simulink model "SimulinkModel"  (R2025b)
settings: Solver=VariableStepAuto  StartTime=0.0  StopTime=90  FixedStep=0.10  MaxStep=0.1  MinStep=0.01  RelTol=0.5e-5  AbsTol=1e-5
values from neighbouring files (symbols this model uses):
  clock_drift_rate = 0.5    [run_simulink_batch.m]
  initial_q_IB = mission.Satellite.q0    [run_simulink_batch.m]
  nav_mekf_initial_P = [1e-2; 1e-2; 1e-2]    [run_simulink_batch.m]
  pod_kf_initial_P = [1e2; 1e2; 1e2; 1e2; 1e2; 1e2]    [run_simulink_batch.m]
  R_mag = diag([1; 2; 3])    [run_simulink_batch.m]
  R_sun = diag([1; 2; 3])    [run_simulink_batch.m]
  s = struct()    [applySensorNoise.m]
  w_earth = [0; 0; 7.2921159 * 10^(-5)]    [run_simulink_batch.m]
undefined symbols (not defined in the file or in its folder): accelCorrectionInterval, baroCorrectionInterval, deg, gpsCorrectionInterval, IAU, IMUPropInterval, magCorrectionInterval, R_vec, rad, WMM2025
libraries: aerolibtransform2 x11, matrix_library x6, vrlib x3, aerolibgravity2 x3, aerolibconvert2 x2, aerolibsatdyn x1, aerolibutil x1, aerolibnav x1
(part 2 of 2)

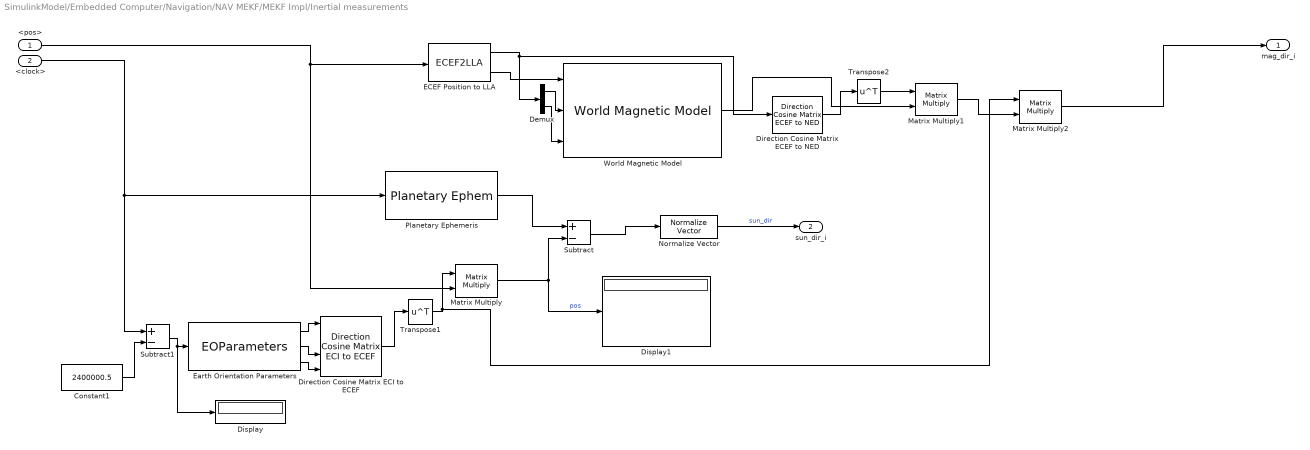
== system SimulinkModel/Embedded Computer/Navigation/NAV MEKF/MEKF Impl/Inertial measurements ==
  <pos> : Inport
  <clock> : Inport  Port=2
  Constant1 : Constant  Value=2400000.5
  Demux : Demux  Outputs=2
  Direction Cosine Matrix ECEF to NED : aerolibtransform2/Direction Cosine Matrix ECEF to NED
  Direction Cosine Matrix ECI to ECEF : aerolibtransform2/Direction Cosine Matrix ECI to ECEF  red=IAU-2000/2006  year=mission.StartDate.Year  month=January  day=1  hour=12  min=0  sec=0  deltaT=None  errorflag=Error  extraparamflag=on
      settings: AttributesFormatString=%<red>
  Display : Display
  Display1 : Display
  ECEF Position to LLA : ECEF2LLA
  Earth Orientation Parameters : EOParameters
  Matrix Multiply : Product  Multiplication=Matrix(*)
  Matrix Multiply1 : Product  Multiplication=Matrix(*)
  Matrix Multiply2 : Product  Multiplication=Matrix(*)
  Normalize Vector : vrlib/Utilities/Normalize Vector  maxzero=0
  Planetary Ephemeris : PlanetaryEphem  units=m,m/s  target=Sun  outputVelocity=off
  Subtract : Sum  Inputs=+-
  Subtract1 : Sum  Inputs=+-
  Transpose1 : Math  Operator=transpose
  Transpose2 : Math  Operator=transpose
  World Magnetic Model : aerolibgravity2/World Magnetic Model  model=WMM2025 (2025-2030)  customFile='WMM2025.COF'  units=Metric (MKS)  time_in=off  month=January  day=1  year=2025  action=Error  h_out=off  dec_out=off  inc_out=off  ti_out=off
  mag_dir_i : Outport
  sun_dir_i : Outport  Port=2
  wires:
  World Magnetic Model/1 -> Matrix Multiply1/2
  <pos>/1 -> Matrix Multiply/2, ECEF Position to LLA/1
  Direction Cosine Matrix ECI to ECEF/1 -> Transpose1/1
  Earth Orientation Parameters/3 -> Direction Cosine Matrix ECI to ECEF/4
  Subtract1/1 -> Display/1, Earth Orientation Parameters/1
  ECEF Position to LLA/1 -> Direction Cosine Matrix ECEF to NED/1, Demux/1
  <clock>/1 -> Planetary Ephemeris/1, Subtract1/1
  Demux/2 -> World Magnetic Model/3
  ECEF Position to LLA/2 -> World Magnetic Model/1
  Earth Orientation Parameters/2 -> Direction Cosine Matrix ECI to ECEF/3
  Earth Orientation Parameters/1 -> Direction Cosine Matrix ECI to ECEF/1
  Transpose1/1 -> Matrix Multiply2/1, Matrix Multiply/1
  Direction Cosine Matrix ECEF to NED/1 -> Transpose2/1
  Transpose2/1 -> Matrix Multiply1/1
  Subtract/1 -> Normalize Vector/1
  Constant1/1 -> Subtract1/2
  Matrix Multiply/1 -> Subtract/2, Display1/1  "pos"
  Demux/1 -> World Magnetic Model/2
  Planetary Ephemeris/1 -> Subtract/1
  Matrix Multiply2/1 -> mag_dir_i/1
  Matrix Multiply1/1 -> Matrix Multiply2/2
  Normalize Vector/1 -> sun_dir_i/1  "sun_dir"

== system SimulinkModel/Embedded Computer/Navigation/NAV MEKF/MEKF Impl/Mag Update ==
  oldState : Inport
  oldP : Inport  Port=2
  <mag> : Inport  Port=3
  mag_i : Inport  Port=4
  Constant : Constant  Value=R_mag
  MATLAB Function : MATLAB Function  TreatAsAtomicUnit=on
  state : Outport
  P : Outport  Port=2
  wires:
  oldState/1 -> MATLAB Function/1(oldState)
  MATLAB Function/1(state) -> state/1
  MATLAB Function/2(P) -> P/1
  oldP/1 -> MATLAB Function/2(oldP)
  <mag>/1 -> MATLAB Function/3(sens)
  Constant/1 -> MATLAB Function/5(R)
  mag_i/1 -> MATLAB Function/4(mag_i)

== system SimulinkModel/Embedded Computer/Navigation/NAV MEKF/MEKF Impl/Sun Update ==
  oldState : Inport
  oldP : Inport  Port=2
  <sun> : Inport  Port=3
  sun_i : Inport  Port=4
  Constant : Constant  Value=R_sun
  MATLAB Function : MATLAB Function  TreatAsAtomicUnit=on
  state : Outport
  P : Outport  Port=2
  wires:
  oldState/1 -> MATLAB Function/1(oldState)
  MATLAB Function/1(state) -> state/1
  MATLAB Function/2(P) -> P/1
  oldP/1 -> MATLAB Function/2(oldP)
  <sun>/1 -> MATLAB Function/3(sens)
  Constant/1 -> MATLAB Function/5(R)
  sun_i/1 -> MATLAB Function/4(sun_i)

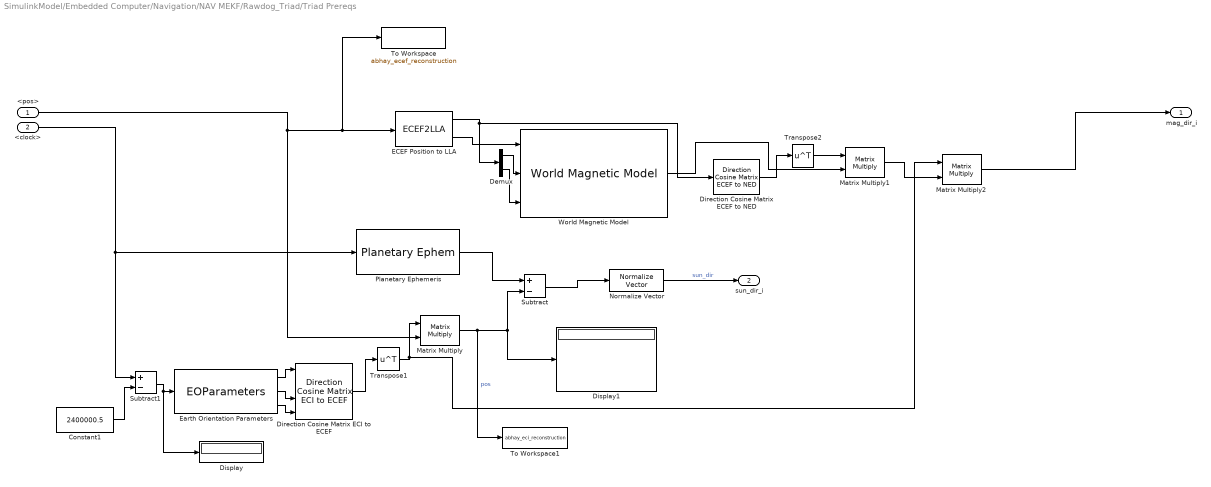
== system SimulinkModel/Embedded Computer/Navigation/NAV MEKF/Rawdog_Triad/Triad Prereqs ==
  <pos> : Inport
  <clock> : Inport  Port=2
  Constant1 : Constant  Value=2400000.5
  Demux : Demux  Outputs=2
  Direction Cosine Matrix ECEF to NED : aerolibtransform2/Direction Cosine Matrix ECEF to NED
  Direction Cosine Matrix ECI to ECEF : aerolibtransform2/Direction Cosine Matrix ECI to ECEF  red=IAU-2000/2006  year=mission.StartDate.Year  month=January  day=1  hour=12  min=0  sec=0  deltaT=None  errorflag=Error  extraparamflag=on
      settings: AttributesFormatString=%<red>
  Display : Display
  Display1 : Display
  ECEF Position to LLA : ECEF2LLA
  Earth Orientation Parameters : EOParameters
  Matrix Multiply : Product  Multiplication=Matrix(*)
  Matrix Multiply1 : Product  Multiplication=Matrix(*)
  Matrix Multiply2 : Product  Multiplication=Matrix(*)
  Normalize Vector : vrlib/Utilities/Normalize Vector  maxzero=0
  Planetary Ephemeris : PlanetaryEphem  units=m,m/s  target=Sun  outputVelocity=off
  Subtract : Sum  Inputs=+-
  Subtract1 : Sum  Inputs=+-
  To Workspace : ToWorkspace  VariableName=abhay_ecef_reconstruction  SaveFormat=Timeseries  SampleTime=-1
  To Workspace1 : ToWorkspace  VariableName=abhay_eci_reconstruction  SaveFormat=Timeseries  SampleTime=-1
  Transpose1 : Math  Operator=transpose
  Transpose2 : Math  Operator=transpose
  World Magnetic Model : aerolibgravity2/World Magnetic Model  model=WMM2025 (2025-2030)  customFile='WMM2025.COF'  units=Metric (MKS)  time_in=off  month=January  day=1  year=2025  action=Error  h_out=off  dec_out=off  inc_out=off  ti_out=off
  mag_dir_i : Outport
  sun_dir_i : Outport  Port=2
  wires:
  World Magnetic Model/1 -> Matrix Multiply1/2
  <pos>/1 -> Matrix Multiply/2, To Workspace/1, ECEF Position to LLA/1
  Direction Cosine Matrix ECI to ECEF/1 -> Transpose1/1
  Earth Orientation Parameters/3 -> Direction Cosine Matrix ECI to ECEF/4
  Subtract1/1 -> Display/1, Earth Orientation Parameters/1
  ECEF Position to LLA/1 -> Direction Cosine Matrix ECEF to NED/1, Demux/1
  <clock>/1 -> Planetary Ephemeris/1, Subtract1/1
  Demux/2 -> World Magnetic Model/3
  ECEF Position to LLA/2 -> World Magnetic Model/1
  Earth Orientation Parameters/2 -> Direction Cosine Matrix ECI to ECEF/3
  Earth Orientation Parameters/1 -> Direction Cosine Matrix ECI to ECEF/1
  Transpose1/1 -> Matrix Multiply2/1, Matrix Multiply/1
  Direction Cosine Matrix ECEF to NED/1 -> Transpose2/1
  Transpose2/1 -> Matrix Multiply1/1
  Subtract/1 -> Normalize Vector/1
  Constant1/1 -> Subtract1/2
  Matrix Multiply/1 -> To Workspace1/1, Subtract/2, Display1/1  "pos"
  Demux/1 -> World Magnetic Model/2
  Planetary Ephemeris/1 -> Subtract/1
  Matrix Multiply2/1 -> mag_dir_i/1
  Matrix Multiply1/1 -> Matrix Multiply2/2
  Normalize Vector/1 -> sun_dir_i/1  "sun_dir"

== matlab function SimulinkModel/Embedded Computer/Navigation/Example Q-Mekf/Gravity/Grav -> Normal force ==
  data: u input; y output
function y = fcn(u)

y = [u(1); u(2); -1.0 * u(3)];

== matlab function SimulinkModel/Embedded Computer/Navigation/Example Q-Mekf/MATLAB Function ==
  data: oldState input; accel_sens input; mag_sens input; gps_sens input; baro_sens input; igrm_model input; state output; P output; use_accel input; oldP input
function [state, P] = fcn(oldState, accel_sens, mag_sens, gps_sens, baro_sens, igrm_model, use_accel, oldP)


%if use_accel
    %[residual, H, R] = measAccelMag(oldState, accel_sens, mag_sens, gps_sens, baro_sens, igrm_model);
%else
    %[residual, H, R] = measMag(oldState, mag_sens, gps_sens, baro_sens, igrm_model);

%end

%disp("Use accel")
%use_accel
%disp("Residual")
%if size(residual, 1) == 2
%residual

%[state, P] = EKFCalculationsAndErrorInject(residual, H, oldP, R, oldState);

state = oldState;
P = oldP;

== matlab function SimulinkModel/Embedded Computer/Navigation/Example Q-Mekf/Mag Update/MATLAB Function ==
  data: oldState input; oldP input; state output; mag_sens input; igrm_model input; R_vec input; P output; oldlastCalcTimes input; magCorrectionInterval input; clock input; lastCalcTimes output
function [state, P, lastCalcTimes] = fcn(oldState, oldP, mag_sens, igrm_model, R_vec, oldlastCalcTimes, magCorrectionInterval, clock)
lastCalcTimes = oldlastCalcTimes;
if clock - oldlastCalcTimes(3) >= magCorrectionInterval

    q = oldState(1:4)';
    
    H_mag = [skewSymmetric(quat2dcm(q) * igrm_model), zeros(3), zeros(3), zeros(3), zeros(3), eye(3), zeros(3, 1)];
    
    h_mag = quat2dcm(q) * igrm_model;
    
    R = diag(R_vec(4:6));
    
    [state, P] = residualErrorInject(oldState, oldP, mag_sens, H_mag, h_mag, R);
else
    state = oldState;
    P = oldP;
end

== matlab function SimulinkModel/Embedded Computer/Navigation/Example Q-Mekf/Unbias sensors/Remove Sensor Bias ==
  data: gyro_sens input; accel_sens input; unbiased_gyro output; unbiased_accel output; mag_sens input; gps_sens input; baro_sens input; state input; unbiased_mag output; unbiased_gps output; unbiased_baro output
function [unbiased_gyro, unbiased_accel, unbiased_mag, unbiased_gps, unbiased_baro] = fcn(gyro_sens, accel_sens, mag_sens, gps_sens, baro_sens, state)

unbiased_gyro = gyro_sens - state(11:13);
unbiased_accel = accel_sens - state(14:16);
unbiased_mag = mag_sens - state(17:19);
unbiased_gps = gps_sens;
unbiased_baro = baro_sens - state(20);



%unbiased_gyro = gyro_sens;
%unbiased_mag = mag_sens;
%unbiased_accel = accel_sens;
%unbiased_baro = baro_sens;

== matlab function SimulinkModel/Embedded Computer/Navigation/Example Q-Mekf/prioriUpdate/EKF Predict ==
  data: prioriState input; P output; gyro_meas input; accel_meas input; oldP input; clock input; lastCalcTimes input; accelCorrectionInterval input; magCorrectionInterval input; gpsCorrectionInterval input; baroCorrectionInterval input
function P = fcn(prioriState, gyro_meas, accel_meas, oldP, clock, lastCalcTimes, accelCorrectionInterval, magCorrectionInterval, gpsCorrectionInterval, baroCorrectionInterval)

if clock - lastCalcTimes(2) > accelCorrectionInterval || clock - lastCalcTimes(3) > magCorrectionInterval || clock - lastCalcTimes(4) > gpsCorrectionInterval || clock - lastCalcTimes(5) > baroCorrectionInterval
    dt = clock - max(lastCalcTimes(2:5));

    stateTransitionMatrix = createProcessModel(prioriState, gyro_meas, accel_meas, dt);
    
    Q_d = createProcessNoise(dt);
    
    P = stateTransitionMatrix * oldP * transpose(stateTransitionMatrix) + Q_d;
else
    P = oldP;
end

== matlab function SimulinkModel/Embedded Computer/Navigation/Example Q-Mekf/prioriUpdate/priori Predict ==
  data: gyro_meas input; newState output; accel_meas input; prevState input; g_i input; lastCalcTimesOld input; clock input; imuPropInterval input; lastCalcTimes output
function [newState, lastCalcTimes] = fcn(gyro_meas, accel_meas, prevState, g_i, lastCalcTimesOld, clock, imuPropInterval)
lastCalcTimes = lastCalcTimesOld;

if clock - lastCalcTimesOld(1) > imuPropInterval
    dt = clock - max(lastCalcTimesOld);
    newState = prioriPropagation(gyro_meas, accel_meas, dt, prevState, g_i);
    lastCalcTimes(1) = clock;
else
    newState = prevState;
end

== matlab function SimulinkModel/Embedded Computer/Navigation/Example Q-Mekf/Accel Update/MATLAB Function ==
  data: oldState input; oldP input; state output; accel_sens input; normal_force input; R_vec input; P output; RocketState input; accelCorrectionInterval input; clock input; lastCalcTimesOld input; lastCalcTimes output
function [state, P, lastCalcTimes] = fcn(oldState, oldP, accel_sens, normal_force, R_vec, RocketState, accelCorrectionInterval, clock, lastCalcTimesOld)

% TODO: One day model the accelerometer using drag forces, etc.
q = oldState(1:4)';
lastCalcTimes = lastCalcTimesOld;

if RocketState == 0 && clock - accelCorrectionInterval >= lastCalcTimesOld(2)
    H_accel = [skewSymmetric(quat2dcm(q) * normal_force), zeros(3), zeros(3), zeros(3), eye(3), zeros(3), zeros(3, 1)];
    
    h_accel = quat2dcm(q) * normal_force;
    
    R = diag(R_vec(1:3));
    
    [state, P] = residualErrorInject(oldState, oldP, accel_sens, H_accel, h_accel, R);
else
    state = oldState;
    P = oldP;
end

== matlab function SimulinkModel/Embedded Computer/Navigation/ODKF/ODKF Impl/EKF Predict ==
  data: state input; P output; oldP input; dt input
function P = fcn(state, oldP, dt)

mu = 3.986004418e14;

pos_norm = norm(state(1:3));


G = [(mu / pos_norm^5) * (3.0 * state(1)^2 - pos_norm^2), 3 * mu * state(1) * state(2) / pos_norm^5, 3 * mu * state(1) * state(3) / pos_norm^5;
    3 * mu * state(1) * state(2) / pos_norm^5, (mu / pos_norm^5) * (3.0 * state(2)^2 - pos_norm^2), 3 * mu * state(2) * state(3) / pos_norm^5;
    3 * mu * state(1) * state(3) / pos_norm^5, 3 * mu * state(2) * state(3) / pos_norm^5, (mu / pos_norm^5) * (3.0 * state(3)^2 - pos_norm^2)];


F = [zeros(3, 3), eye(3, 3); G, zeros(3, 3)];

tuning_param_var = 1e-1;

Q_d = tuning_param_var * [(dt^3 / 3.0) * eye(3), (dt^2 / 2.0) * eye(3); (dt^2 / 2.0) * eye(3), dt * eye(3)];


phi = eye(6) + F * dt;

P = phi * oldP * phi' + Q_d;

== matlab function SimulinkModel/Embedded Computer/Navigation/ODKF/ODKF Impl/EKF Update ==
  data: oldState input; state output; oldP input; P output; meas input
function [state, P] = fcn(oldState, oldP, meas)

H = eye(6);

R = diag([2^2; 2^2; 2^2; 0.5^2; 0.5^2; 0.5^2]);

S = H * oldP * H' + R;

K = (oldP * H') / S;

state = oldState + K * (meas - oldState);

P = (eye(6) - K * H) * oldP * (eye(6) - K * H)' + K * R * K';

== matlab function SimulinkModel/Embedded Computer/Navigation/NAV MEKF/MEKF Impl/Gyro Prop ==
  data: oldState input; state output; gyro_meas input; dt input
function state = fcn(oldState, gyro_meas, dt)

state = oldState;

rot_vec = 1.0 * gyro_meas * dt;

q = oldState(1:4)';


rot_vec_norm = norm(rot_vec);
axis = rot_vec / rot_vec_norm;

if min(rot_vec_norm) < 1e-9 % Small angle approx if small angle
    dq = [1; 0.5*rot_vec];
else
    dq = [cos(rot_vec_norm / 2.0); (axis * sin(rot_vec_norm / 2.0))]';
end

q = quatmultiply(q, dq);
q = q / norm(q);

state(1:4) = q';

== matlab function SimulinkModel/Embedded Computer/Navigation/NAV MEKF/Rawdog_prop/MATLAB Function ==
  data: oldState input; state output; gyro_meas input; dt input
function state = fcn(oldState, gyro_meas, dt)

state = oldState;

rot_vec = 1.0 * gyro_meas * dt;

q = oldState(1:4)';


rot_vec_norm = norm(rot_vec);
axis = rot_vec / rot_vec_norm;

if min(rot_vec_norm) < 1e-9 % Small angle approx if small angle
    dq = [1; 0.5*rot_vec];
else
    dq = [cos(rot_vec_norm / 2.0); (axis * sin(rot_vec_norm / 2.0))]';
end

q = quatmultiply(q, dq);
q = q / norm(q);

state(1:4) = q';

== matlab function SimulinkModel/Embedded Computer/Navigation/NAV MEKF/Rawdog_Triad/MATLAB Function ==
  data: R_IB output; v_1b input; v_2b input; v_1i input; v_2i input
function R_IB = fcn(v_1b, v_2b, v_1i, v_2i)

R_IB = triad(v_1b, v_2b, v_1i, v_2i);

== matlab function SimulinkModel/Embedded Computer/Navigation/NAV MEKF/MEKF Impl/EKF Pred ==
  data: oldState input; gyro_meas input; oldP input; P output; dt input
function P = fcn(oldState, gyro_meas, oldP, dt)

phi = createProcessModel(oldState, gyro_meas, dt);

Q = createProcessNoise(dt);

P = phi * oldP * phi' + Q;

== matlab function SimulinkModel/Embedded Computer/Navigation/NAV MEKF/Rawdog_Triad/dummy_func ==
  data: oldClock input; clock output; dt input
function clock = fcn(oldClock, dt)

clock = oldClock;

== matlab function SimulinkModel/Embedded Computer/Navigation/NAV MEKF/MEKF Impl/Mag Update/MATLAB Function ==
  data: oldState input; oldP input; sens input; mag_i input; R input; state output; P output
function [state, P] = fcn(oldState, oldP, sens, mag_i, R)

H = skewSymmetric(quat2dcm(oldState(1:4)') * mag_i);

h = quat2dcm(oldState(1:4)') * mag_i;

[state, P] = residualErrorInject(oldState, oldP, sens, H, h, R);

== matlab function SimulinkModel/Embedded Computer/Navigation/NAV MEKF/MEKF Impl/Sun Update/MATLAB Function ==
  data: oldState input; oldP input; sens input; sun_i input; R input; state output; P output
function [state, P] = fcn(oldState, oldP, sens, sun_i, R)

H = skewSymmetric(quat2dcm(oldState(1:4)') * sun_i);

h = quat2dcm(oldState(1:4)') * sun_i;

[state, P] = residualErrorInject(oldState, oldP, sens, H, h, R);

== matlab function SimulinkModel/Embedded Computer/Sensors/Create Sun Sensor/MATLAB Function ==
  data: norm_pos_i input; sun_body output; q_IB input; sun_body input
function sun_body = fcn(norm_pos_i, q_IB, sun_body)

roll_axis_body = [1; 0; 0];

roll_axis_inertial = quat2rotm(q_IB) * roll_axis_body;

theta = acos((norm_pos_i * roll_axis_inertial));

if theta > deg2rad(60)
    sun_body = [0; 0; 0];
end

== matlab function SimulinkModel/Embedded Computer/Navigation/Example Q-Mekf/Baro Update/MATLAB Function ==
  data: oldState input; height input; oldP input; state output; baro_sens input; R_vec input; P output; oldlastCalcTimes input; baro_correction_interval input; clock input; lastCalcTimes output
function [state, P, lastCalcTimes] = fcn(oldState, height, oldP, baro_sens, R_vec, oldlastCalcTimes, baro_correction_interval, clock)
% TODO subject of future research
%if clock - lastCalcTimes(4) >= gps_correction_interval
% TODO these are here b/c I don't know how to matlab, otherwise erase
P0 = 101325;
L  = 0.0065;
T0  = 288.15;
M   = 0.0289644;
R   = 8.3144598;
g_e = 9.80665;

H_baro = [zeros(1, 3), zeros(1, 3), [0, 0, 0], zeros(1, 3), zeros(1, 3), zeros(1, 3), 1];

h_baro = P0 * (1 - (L * height) / T0)^(g_e*M / (R*L));

%disp("Recreation of baro")
%disp(h_baro)
%disp("Actual baro")
%disp(baro_sens)

R = R_vec(10);

[state, P] = residualErrorInject(oldState, oldP, baro_sens, H_baro, h_baro, R);

== stateflow chart SimulinkModel/Embedded Computer/State Machine/Chart ==
  data: data input; data1 output

== matlab function SimulinkModel/Embedded Computer/Sensors/MATLAB Function ==
  data: jd input; new_jd output; startDate input; clock_drift_rate input
function new_jd = fcn(jd, startDate, clock_drift_rate)
    curr_dt = datetime(jd,'convertfrom','juliandate');
    elapsed_time = curr_dt - startDate;
    new_dt = DAY(elapsed_time) + days(elapsed_time) * clock_drift_rate;
    new_jd = juliandate(new_dt);

== matlab function SimulinkModel/Embedded Computer/Navigation/ODKF/ODKF Impl/RK4 Propate ==
  data: state input; new_state output; dt input
function new_state = fcn(state, dt)

k1 = get_step(state);
k2 = get_step(state + (dt / 2.0) * k1);
k3 = get_step(state + (dt / 2.0) * k2);
k4 = get_step(state + dt * k3);
new_state = state + (dt / 6.0) * (k1 + 2 * k2 + 2 * k3 + k4);

== matlab function SimulinkModel/Dynamics/Diff from ITA to UTC   ==
  data: year input; tai_utc_diff output; month input; day input; hour input; minute input; second input
function tai_utc_diff = calculateTAI_UTC(year, month, day, hour, minute, second) 
    % List of leap seconds added to UTC since 1972 
    leap_seconds = { 
        datetime(1972, 7, 1), 10; 
        datetime(1973, 1, 1), 11; 
        datetime(1974, 1, 1), 12; 
        datetime(1975, 1, 1), 13; 
        datetime(1976, 1, 1), 14; 
        datetime(1977, 1, 1), 15; 
        datetime(1978, 1, 1), 16; 
        datetime(1979, 1, 1), 17; 
        datetime(1980, 1, 1), 18; 
        datetime(1981, 7, 1), 19; 
        datetime(1982, 7, 1), 20; 
        datetime(1983, 7, 1), 21; 
        datetime(1985, 7, 1), 22; 
        datetime(1988, 1, 1), 23; 
        datetime(1990, 1, 1), 24; 
        datetime(1991, 1, 1), 25; 
        datetime(1992, 7, 1), 26; 
        datetime(1993, 7, 1), 27; 
        datetime(1994, 7, 1), 28; 
        datetime(1996, 1, 1), 29; 
        datetime(1997, 7, 1), 30; 
        datetime(1999, 1, 1), 31; 
        datetime(2006, 1, 1), 32; 
        datetime(2009, 1, 1), 33; 
        datetime(2012, 7, 1), 34; 
        datetime(2015, 7, 1), 35; 
        datetime(2017, 1, 1), 36; 
        datetime(2023, 1, 1), 37; 
    }; 
    % Create a datetime object for the input date 
    input_date = datetime(year, month, day, hour, minute, second); 
    % Initialize TAI-UTC difference 
    tai_utc_diff = 10; 
    % Loop through leap seconds and find the applicable difference 
    for i = 1:size(leap_seconds, 1) 
        if input_date >= leap_seconds{i, 1} 
            tai_utc_diff = leap_seconds{i, 2}; 
        else
            break; 
        end 
    end
end 

% Example: Calculate TAI-UTC difference for January 1, 2024, at 12:00:00 
diff = calculateTAI_UTC(2024, 1, 1, 12, 0, 0); 
fprintf('TAI-UTC difference: %d seconds\n', diff);

== matlab function SimulinkModel/Embedded Computer/Sensors/Create Mag/corrupt_mag ==
  data: oldMag input; mag output
function mag = fcn(oldMag)

mag = oldMag;

== matlab function SimulinkModel/Embedded Computer/Navigation/Example Q-Mekf/GPS Update/MATLAB Function ==
  data: oldState input; oldP input; state output; gps_sens input; R_vec input; P output; oldlastCalcTimes input; gps_correction_interval input; clock input; lastCalcTimes output
function [state, P, lastCalcTimes] = fcn(oldState, oldP, gps_sens, R_vec, oldlastCalcTimes, gps_correction_interval, clock)

lastCalcTimes = oldlastCalcTimes;

if clock - lastCalcTimes(4) >= gps_correction_interval

    H_gps = [zeros(3), zeros(3), eye(3), zeros(3), zeros(3), zeros(3), zeros(3, 1)];
    
    h_gps = oldState(8:10);
    
    R = diag(R_vec(7:9));
    
    [state, P] = residualErrorInject(oldState, oldP, gps_sens, H_gps, h_gps, R);
else
    state = oldState;
    P = oldP;
end
